simulink model "ADAS_Main_ClosedLoop"  (R2026a)
settings: Solver=FixedStepDiscrete  StopTime=20
InitFcn:
  | createLidarActorProfiles;
  | % L3/L4 closed-loop ego initial condition, READ FROM THE TEST-1 FIXTURE
  | % (not hard-coded in the vehicle model, which stays reusable)
  | clS = load('D:\AutonomousDriving\D_scenarios\V2_0_ClosedLoop_Test9_TwoObstacles_WideRoad.mat');
  | clA = clS.data.ActorSpecifications([clS.data.ActorSpecifications.ActorID] == clS.data.EgoCarId);
  | CL_EGO_IC = [clA.Position(1); clA.Position(2); clA.Yaw*pi/180; clA.Speed(1)];
  | clear clS clA
  | % Non-virtual ego-pose bus type. A MATLAB Function block (Extract_Ego_Kinematics)
  | % cannot accept a VIRTUAL bus, so the Bus Creator must emit a defined Simulink.Bus.
  | % Shape copied from the installed validator contract and from BusActorsActors.
  | clN = {'ActorID','Position','Velocity','Roll','Pitch','Yaw','AngularVelocity'};
  | clD = {[1 1],[1 3],[1 3],[1 1],[1 1],[1 1],[1 3]};
  | clEls = Simulink.BusElement.empty(0,1);
  | for clI = 1:7
  |   clE = Simulink.BusElement; clE.Name = clN{clI}; clE.Dimensions = clD{clI}; clE.DataType = 'double';
  |   clEls(clI,1) = clE;
  | end
  | BusEgoPose_CL = Simulink.Bus; BusEgoPose_CL.Elements = clEls;
  | clear clN clD clEls clE clI
StopFcn:
  | cl_plot_closedloop_trajectory;
model workspace (MAT data in the model file):
  firstWarning = 1
  originalScenarioChecksum = '71EAF3DF157DF5A35F75811B676F8B0F'
undefined symbols (not defined in the file): driving, matlabshared
libraries: drivingscenarioandsensors x3, lidarlib x1
(part 3 of 7)

== matlab function ADAS_Main_ClosedLoop/Tracking_Prediction/Track_Association ==
  data: trkState input; trkAssign output; trkCov input; trkID input; trkStatus input; fusedObjects input; numFusedObjects input; numAssigned output; assocDiag output
function [trkAssign, numAssigned, assocDiag] = Track_Association( ...
    trkState, trkCov, trkID, trkStatus, fusedObjects, numFusedObjects)
%#codegen
% TRACK_ASSOCIATION  Stage 3: measurement-to-track association ONLY.
%
% THIS BLOCK DOES NOT: update track state, create tracks, confirm, coast,
% delete, run any lifecycle, keep history, or emit prediction horizons.
% It is a PURE FUNCTION of the predicted tracks and the current detections -
% it holds no state and has no Unit Delay. Track Update is a later stage.
%
% PIPELINE
%   Mahalanobis gating -> connected components -> Munkres (max(m,n) <= 32)
%                      -> deterministic greedy-by-cost fallback otherwise
%
% MAX_COMPONENT NOTE (flagged, not silently chosen): the frozen text says both
% "components <= 32 total nodes" and "L = m + n, maximum matrix size 64 x 64".
% Those are inconsistent - m+n <= 32 implies a 32x32 matrix. The 64x64
% allocation follows only from max(m,n) <= 32, which is also the definition the
% measured component statistics used. This implementation bounds max(m,n) <= 32
% and allocates 64x64, which is STRICTLY MORE CAPABLE: every component with
% m+n <= 32 is still solved exactly by Munkres.
%
% INNOVATION COVARIANCE
%   S = H*Ppred*H' + R + W ,  H selects [X Y] ,  W = SIGMA_W^2 * I
%   R is the detection's FULL 2x2 fused position covariance, used as-is.
%   W is applied ONLY here, never in Q. The LiDAR reference-point D^2/12 term is
%   NOT re-applied - Sensor Fusion already incorporated it into R.
%   The full 2x2 is used: never scalarised, never clamped, no axis-aligned box.
%
%   d2 = r' * inv(S) * r   via the validated analytic 2x2 inverse with a
%   positive-definiteness guard. Never inv(), never Inf/NaN sentinels.
%   Gated iff d2 <= CHI2_GATE.
%
% DETERMINISM
%   Component members are insertion-sorted by (TrackID, slot index) for tracks
%   and by index for detections BEFORE the cost matrix is built, so Munkres'
%   ascending scans implement the frozen tie-break: cost -> TrackID -> detection
%   index. Slot index is never used as identity.
%
% OUTPUT  trkAssign [512 x 7], row = track slot
%   1 Assigned      1 if this slot holds an active track with an assignment
%   2 TrackID       persistent identity (0 while none has been allocated)
%   3 DetIdx        1-based row in fusedObjects; 0 = unassigned
%   4 Cost          Mahalanobis d2 of the assignment
%   5 Margin        second-best gated cost - assigned cost; BIG if uncontested
%   6 Flags         1 SuboptimalAssignment | 2 DisplacedAssignment
%                   4 LowMargin (< MARGIN_MIN) | 8 Uncontested
%                   16 HadGatedCandidate      | 32 IterationCapHit
%   7 ComponentSize max(nTracks, nDets) of the component this track was in
%
%   MARGIN_MIN IS A DIAGNOSTIC ONLY. A low or negative margin NEVER rejects,
%   deletes or invalidates an assignment.
%
% assocDiag [1 x 8]
%   1 nActiveTracks   2 nValidDetections  3 nCandidates   4 nComponents
%   5 maxComponentSize 6 nFallbackComponents 7 candidateOverflow 8 nCovRejected
%
% SCENARIO INDEPENDENCE: consumes only predicted track state and fused
% detections. No actor identity, class, count, trajectory, map or scenario
% geometry. Loop bounds are the declared interface capacities.

MAX_T    = 512;
MAX_D    = 356;
MAX_C    = 8192;
MAX_COMP = 32;
MAX_L    = 64;

CHI2_GATE  = 9.21;
SIGMA_W    = 0.40;
WVAR       = SIGMA_W*SIGMA_W;
BIG        = 1e9;
DUMMY      = 9.21;
MARGIN_MIN = 2.0;

C_VALID = 1; C_X = 2; C_Y = 3; C_CXX = 5; C_CYY = 6; C_CXY = 7;

trkAssign   = zeros(MAX_T, 7);
numAssigned = uint32(0);
assocDiag   = zeros(1, 8);

nD = double(numFusedObjects);
if nD < 0,     nD = 0;     end
if nD > MAX_D, nD = MAX_D; end

% ---- 1. active tracks and valid detections -------------------------------
trkActive = false(MAX_T,1);
nAct = 0;
for t = 1:MAX_T
    trkAssign(t,2) = double(trkID(t));
    if trkStatus(t) ~= 0
        trkActive(t) = true;
        nAct = nAct + 1;
    end
end
detValid = false(MAX_D,1);
nDet = 0;
for j = 1:nD
    if fusedObjects(j,C_VALID) == 1
        detValid(j) = true;
        nDet = nDet + 1;
    end
end
assocDiag(1) = nAct;
assocDiag(2) = nDet;

if nAct == 0 || nDet == 0
    return                       % nothing to associate - deterministic no-op
end

% ---- 2. gating -----------------------------------------------------------
gate  = false(MAX_T, MAX_D);
cand  = zeros(MAX_C, 3);         % cost, trackSlot, detIdx
nCand = 0;
ovf   = 0;
nCovRej = 0;
bestC = zeros(MAX_T,1);          % best gated cost per track
best2 = zeros(MAX_T,1);          % second-best gated cost per track
for t = 1:MAX_T
    bestC(t) = BIG; best2(t) = BIG;
end

for t = 1:MAX_T
    if ~trkActive(t), continue; end
    p11 = trkCov(t,1); p12 = trkCov(t,2); p22 = trkCov(t,5);
    xh  = trkState(t,1); yh = trkState(t,2);
    for j = 1:nD
        if ~detValid(j), continue; end
        s11 = p11 + fusedObjects(j,C_CXX) + WVAR;
        s22 = p22 + fusedObjects(j,C_CYY) + WVAR;
        s12 = p12 + fusedObjects(j,C_CXY);
        if ~isPD2(s11, s22, s12)
            nCovRej = nCovRej + 1;
            continue
        end
        dt_ = s11*s22 - s12*s12;
        dx  = fusedObjects(j,C_X) - xh;
        dy  = fusedObjects(j,C_Y) - yh;
        d2  = (dx*dx*s22 - 2*dx*dy*s12 + dy*dy*s11) / dt_;
        if ~isfinite(d2) || d2 < 0
            nCovRej = nCovRej + 1;
            continue
        end
        if d2 <= CHI2_GATE
            if nCand < MAX_C
                nCand = nCand + 1;
                cand(nCand,1) = d2;
                cand(nCand,2) = t;
                cand(nCand,3) = j;
                gate(t,j) = true;
                if d2 < bestC(t)
                    best2(t) = bestC(t);
                    bestC(t) = d2;
                elseif d2 < best2(t)
                    best2(t) = d2;
                end
            else
                ovf = 1;
            end
        end
    end
end
assocDiag(3) = nCand;
assocDiag(7) = ovf;
assocDiag(8) = nCovRej;

if nCand == 0
    return
end

% ---- 3. connected components of the bipartite gated graph ---------------
% Same fixed-size union-find pattern already validated in Cluster_BEV.
NN = MAX_T + MAX_D;
par = zeros(NN,1);
for k = 1:NN
    par(k) = k;
end
for c = 1:nCand
    a = cand(c,2);
    b = MAX_T + cand(c,3);
    while par(a) ~= a, a = par(a); end
    while par(b) ~= b, b = par(b); end
    if a ~= b
        if a < b, par(b) = a; else, par(a) = b; end
    end
end
root = zeros(NN,1);
for k = 1:NN
    a = k;
    while par(a) ~= a, a = par(a); end
    root(k) = a;
end

% ---- 4. solve each component --------------------------------------------
compDone = false(NN,1);
nComp = 0; maxComp = 0; nFallback = 0;
asgDet  = zeros(MAX_T,1);
asgCost = zeros(MAX_T,1);
asgFlag = zeros(MAX_T,1);
asgCsz  = zeros(MAX_T,1);
usedT   = false(MAX_T,1);
usedD   = false(MAX_D,1);
mTrk = zeros(MAX_COMP,1);
mDet = zeros(MAX_COMP,1);
Cm   = zeros(MAX_L, MAX_L);

for c = 1:nCand
    rt = root(cand(c,2));
    if compDone(rt), continue; end
    compDone(rt) = true;

    % ---- count members WITHOUT truncating (an oversized component is
    %      solved whole by the fallback, never silently split)
    m = 0; n = 0;
    for t = 1:MAX_T
        if trkActive(t) && root(t) == rt, m = m + 1; end
    end
    for j = 1:nD
        if detValid(j) && root(MAX_T + j) == rt, n = n + 1; end
    end
    if m == 0 || n == 0, continue; end
    nComp = nComp + 1;
    csz = m; if n > csz, csz = n; end
    if csz > maxComp, maxComp = csz; end

    useMunkres = (m <= MAX_COMP) && (n <= MAX_COMP);
    capHit = false;

    if useMunkres
        % ---- gather and order members deterministically
        m = 0; n = 0;
        for t = 1:MAX_T
            if trkActive(t) && root(t) == rt, m = m + 1; mTrk(m) = t; end
        end
        for j = 1:nD
            if detValid(j) && root(MAX_T + j) == rt, n = n + 1; mDet(n) = j; end
        end
        for a = 2:m                      % insertion sort by (TrackID, slot)
            kt = mTrk(a); kid = double(trkID(kt)); b = a - 1; placed = false;
            while b >= 1 && ~placed
                pt = mTrk(b); pid = double(trkID(pt));
                if (pid > kid) || (pid == kid && pt > kt)
                    mTrk(b+1) = mTrk(b); b = b - 1;
                else
                    placed = true;
                end
            end
            mTrk(b+1) = kt;
        end
        for a = 2:n                      % insertion sort by index
            kd = mDet(a); b = a - 1;
            while b >= 1 && mDet(b) > kd
                mDet(b+1) = mDet(b); b = b - 1;
            end
            mDet(b+1) = kd;
        end

        L = m + n;
        for a = 1:L
            for b = 1:L
                Cm(a,b) = BIG;
            end
        end
        for a = 1:m
            Cm(a, n+a) = DUMMY;
        end
        for b = 1:n
            Cm(m+b, b) = DUMMY;
            for a = 1:m
                Cm(m+b, n+a) = 0;
            end
        end
        for cc = 1:nCand
            ts = cand(cc,2);
            if root(ts) ~= rt, continue; end
            ds = cand(cc,3);
            ai = 0; bi = 0;
            for a = 1:m
                if mTrk(a) == ts, ai = a; break; end
            end
            for b = 1:n
                if mDet(b) == ds, bi = b; break; end
            end
            if ai > 0 && bi > 0, Cm(ai,bi) = cand(cc,1); end
        end

        [asgL, capHit] = munkres_fixed(Cm, L, MAX_L);
        if ~capHit
            for a = 1:m
                b = asgL(a);
                if b >= 1 && b <= n
                    t = mTrk(a); j = mDet(b);
                    asgDet(t) = j; asgCsz(t) = csz;
                    for cc = 1:nCand
                        if cand(cc,2) == t && cand(cc,3) == j
                            asgCost(t) = cand(cc,1); break
                        end
                    end
                end
            end
        else
            useMunkres = false;
        end
    end

    if ~useMunkres
        % ---- deterministic greedy-by-cost over the WHOLE component.
        % Scans the candidate list directly, so an oversized component is
        % solved entire - it is never split or truncated.
        nFallback = nFallback + 1;
        nPick = m; if n < nPick, nPick = n; end
        for pick = 1:nPick
            bc = BIG; bt = 0; bd = 0; bid = 0;
            for cc = 1:nCand
                t = cand(cc,2);
                if root(t) ~= rt, continue; end
                j = cand(cc,3);
                if usedT(t) || usedD(j), continue; end
                cv = cand(cc,1); tid = double(trkID(t));
                take = false;
                if cv < bc
                    take = true;
                elseif cv == bc
                    if tid < bid
                        take = true;
                    elseif tid == bid && j < bd
                        take = true;
                    end
                end
                if take
                    bc = cv; bt = t; bd = j; bid = tid;
                end
            end
            if bt == 0, break; end
            usedT(bt) = true; usedD(bd) = true;
            asgDet(bt) = bd; asgCost(bt) = bc; asgCsz(bt) = csz;
            asgFlag(bt) = asgFlag(bt) + 1;                 % SuboptimalAssignment
            if capHit, asgFlag(bt) = asgFlag(bt) + 32; end % IterationCapHit
        end
    end
end
assocDiag(4) = nComp;
assocDiag(5) = maxComp;
assocDiag(6) = nFallback;

% ---- 5. write results, margins and flags --------------------------------
nAsg = 0;
for t = 1:MAX_T
    if ~trkActive(t), continue; end
    fl = asgFlag(t);
    if bestC(t) < BIG, fl = fl + 16; end          % HadGatedCandidate
    j = asgDet(t);
    if j > 0
        nAsg = nAsg + 1;
        ac = asgCost(t);
        alt = BIG;
        for cc = 1:nCand
            if cand(cc,2) == t && cand(cc,3) ~= j
                if cand(cc,1) < alt, alt = cand(cc,1); end
            end
        end
        if alt >= BIG
            mg = BIG;
            fl = fl + 8;                          % Uncontested
        else
            mg = alt - ac;
            if mg < 0,          fl = fl + 2; end  % DisplacedAssignment
            if mg < MARGIN_MIN, fl = fl + 4; end  % LowMargin (DIAGNOSTIC ONLY)
        end
        trkAssign(t,1) = 1;
        trkAssign(t,3) = j;
        trkAssign(t,4) = ac;
        trkAssign(t,5) = mg;
    else
        trkAssign(t,5) = BIG;
    end
    trkAssign(t,6) = fl;
    trkAssign(t,7) = asgCsz(t);
end
numAssigned = uint32(nAsg);

end

% ===========================================================================
function tf = isPD2(a, b, c)
% 2x2 symmetric [a c; c b] is positive definite iff a > 0 and det > 0.
tf = false;
if isfinite(a) && isfinite(b) && isfinite(c)
    if a > 0 && b > 0 && (a*b - c*c) > 0
        tf = true;
    end
end
end

% ===========================================================================
function [asg, capHit] = munkres_fixed(Cin, L, MAX_L)
% Fixed-size Munkres / Hungarian on the L x L leading block of Cin.
% Iterative (no recursion), no dynamic arrays, no sort/unique, no Inf/NaN.
% Ascending index scans make every tie deterministic; the caller orders the
% component members so this realises cost -> TrackID -> detection index.
% Iteration limit L^2 per the frozen spec; on hit, capHit is set and the caller
% falls back to deterministic greedy.
HUGE = 1e18;
asg    = zeros(MAX_L,1);
capHit = false;
C = zeros(MAX_L,MAX_L);
for i = 1:L
    for j = 1:L
        C(i,j) = Cin(i,j);
    end
end
for i = 1:L
    mn = C(i,1);
    for j = 2:L
        if C(i,j) < mn, mn = C(i,j); end
    end
    for j = 1:L
        C(i,j) = C(i,j) - mn;
    end
end
for j = 1:L
    mn = C(1,j);
    for i = 2:L
        if C(i,j) < mn, mn = C(i,j); end
    end
    for i = 1:L
        C(i,j) = C(i,j) - mn;
    end
end
star = false(MAX_L,MAX_L); prim = false(MAX_L,MAX_L);
rowCov = false(MAX_L,1); colCov = false(MAX_L,1);
rowHas = false(MAX_L,1); colHas = false(MAX_L,1);
path = zeros(2*MAX_L,2);
for i = 1:L
    for j = 1:L
        if C(i,j) == 0 && ~rowHas(i) && ~colHas(j)
            star(i,j) = true; rowHas(i) = true; colHas(j) = true;
        end
    end
end
CAP = L*L; iter = 0; step = 4; zr = 0; zc = 0;
while step ~= 0
    iter = iter + 1;
    if iter > CAP, capHit = true; break; end
    if step == 4
        for j = 1:L, colCov(j) = false; end
        ncov = 0;
        for j = 1:L
            for i = 1:L
                if star(i,j), colCov(j) = true; break; end
            end
            if colCov(j), ncov = ncov + 1; end
        end
        if ncov >= L, step = 0; else, step = 5; end
    elseif step == 5
        zr = 0; zc = 0;
        for i = 1:L
            if rowCov(i), continue; end
            for j = 1:L
                if ~colCov(j) && C(i,j) == 0
                    zr = i; zc = j; break
                end
            end
            if zr > 0, break; end
        end
        if zr == 0
            step = 7;
        else
            prim(zr,zc) = true;
            sc = 0;
            for j = 1:L
                if star(zr,j), sc = j; break; end
            end
            if sc > 0
                rowCov(zr) = true; colCov(sc) = false; step = 5;
            else
                step = 6;
            end
        end
    elseif step == 6
        cnt = 1; path(1,1) = zr; path(1,2) = zc;
        guard = 0; goOn = true;
        while goOn
            guard = guard + 1;
            if guard > CAP, capHit = true; goOn = false; break; end
            rr = 0;
            for i = 1:L
                if star(i,path(cnt,2)), rr = i; break; end
            end
            if rr > 0
                cnt = cnt + 1; path(cnt,1) = rr; path(cnt,2) = path(cnt-1,2);
                cc = 0;
                for j = 1:L
                    if prim(rr,j), cc = j; break; end
                end
                cnt = cnt + 1; path(cnt,1) = rr; path(cnt,2) = cc;
            else
                goOn = false;
            end
        end
        if capHit, break; end
        for k = 1:cnt
            if star(path(k,1),path(k,2))
                star(path(k,1),path(k,2)) = false;
            else
                star(path(k,1),path(k,2)) = true;
            end
        end
        for i = 1:L, rowCov(i) = false; colCov(i) = false; end
        for i = 1:L
            for j = 1:L
                prim(i,j) = false;
            end
        end
        step = 4;
    else
        mn = HUGE;
        for i = 1:L
            if rowCov(i), continue; end
            for j = 1:L
                if ~colCov(j) && C(i,j) < mn, mn = C(i,j); end
            end
        end
        if mn >= HUGE, capHit = true; break; end
        for i = 1:L
            for j = 1:L
                if rowCov(i),  C(i,j) = C(i,j) + mn; end
                if ~colCov(j), C(i,j) = C(i,j) - mn; end
            end
        end
        step = 5;
    end
end
if ~capHit
    for i = 1:L
        for j = 1:L
            if star(i,j), asg(i) = j; break; end
        end
    end
end
end
